simulink model "ex5sim"  (R2017a)
settings: Solver=VariableStepAuto  StartTime=0.0  StopTime=tf  RelTol=1e-3
values from neighbouring files (symbols this model uses):
  x0 = [1, 1]    [ex5scr.m]
settings Model: Creator=bruno  LastModifiedBy=bruno

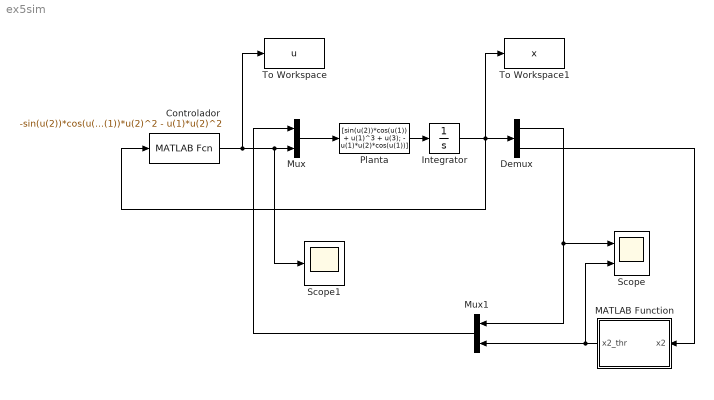
== system ex5sim ==
  Controlador : MATLABFcn  MATLABFcn=-sin(u(2))*cos(u(1)) - u(1)^3 + cos(u(1))*u(2)^2 - u(1)*u(2)^2  OutputDimensions=1
  Demux : Demux  Outputs=2
  Integrator : Integrator  InitialCondition=x0
  MATLAB Function : MATLAB Function  TreatAsAtomicUnit=on
  Mux : Mux  Inputs=2
  Mux1 : Mux  Inputs=2
  Planta : MATLABFcn  MATLABFcn=[sin(u(2))*cos(u(1)) + u(1)^3 + u(3); - u(1)*u(2)*cos(u(1))]  OutputDimensions=2
  Scope : Scope  NumInputPorts=2
  Scope1 : Scope
  To Workspace : ToWorkspace  VariableName=u  SaveFormat=Structure With Time  SampleTime=-1
  To Workspace1 : ToWorkspace  VariableName=x  SaveFormat=Structure With Time  SampleTime=-1
  wires:
  Planta/1 -> Integrator/1
  Controlador/1 -> Scope1/1, Mux/2, To Workspace/1
  Mux/1 -> Planta/1
  Mux1/1 -> Mux/1
  MATLAB Function/1(x2_thr) -> Mux1/2, Scope/2
  Demux/1 -> Scope/1, Mux1/1
  Integrator/1 -> Demux/1, To Workspace1/1, Controlador/1
  Demux/2 -> MATLAB Function/1(x2)

== matlab function ex5sim/MATLAB Function ==
  data: x2 input; x2_thr output
function x2_thr = fcn(x2)
    if((x2 < 1e-3)||(x2 > -1e-3))
        x2_thr = x2;
    else
        x2_thr = 0;
    end
